simulink model "SF104A_MotCurrRegCfg"  (R2013b)
settings: Solver=FixedStepDiscrete  SolverMode=SingleTasking  StartTime=0.0  StopTime=1  FixedStep=0.002  RelTol=1e-3
values from neighbouring files (symbols this model uses):
  ARCHGLBPRM_2MILLISEC_SEC_F32 = DataDict.Constant    [SF104A_MotCurrRegCfg_DataDict.m]
  ARCHGLBPRM_2PI_ULS_F32 = DataDict.Constant    [SF104A_MotCurrRegCfg_DataDict.m]
  ARCHGLBPRM_HALFSQRT3_ULS_F32 = DataDict.Constant    [SF104A_MotCurrRegCfg_DataDict.m]
  MotCurrRegCfgCtrlrDynGainVehSpdCutOff = DataDict.Calibration    [SF104A_MotCurrRegCfg_DataDict.m]
  MotCurrRegCfgCurrLoopSecOrderTrfFctEna = DataDict.Calibration    [SF104A_MotCurrRegCfg_DataDict.m]
  MotCurrRegCfgIntglGainSampleTi = DataDict.Calibration    [SF104A_MotCurrRegCfg_DataDict.m]
  MotCurrRegCfgMotAgCompuDly = DataDict.Calibration    [SF104A_MotCurrRegCfg_DataDict.m]
  MotCurrRegCfgMotClsdLoopBwDaxY = DataDict.Calibration    [SF104A_MotCurrRegCfg_DataDict.m]
  MotCurrRegCfgMotClsdLoopBwQaxY = DataDict.Calibration    [SF104A_MotCurrRegCfg_DataDict.m]
  MotCurrRegCfgMotDampgRatDax = DataDict.Calibration    [SF104A_MotCurrRegCfg_DataDict.m]
  MotCurrRegCfgMotDampgRatQax = DataDict.Calibration    [SF104A_MotCurrRegCfg_DataDict.m]
  MotCurrRegCfgMotNatFrqDaxY = DataDict.Calibration    [SF104A_MotCurrRegCfg_DataDict.m]
  MotCurrRegCfgMotNatFrqQaxY = DataDict.Calibration    [SF104A_MotCurrRegCfg_DataDict.m]
  MotCurrRegCfgMotRVirtDax = DataDict.Calibration    [SF104A_MotCurrRegCfg_DataDict.m]
  MotCurrRegCfgMotRVirtQax = DataDict.Calibration    [SF104A_MotCurrRegCfg_DataDict.m]
  MOTDAMPGRATCON_ULS_F32 = DataDict.Constant    [SF104A_MotCurrRegCfg_DataDict.m]
  MotRefMdlFbCtrlDi = DataDict.ImprtdCal    [SF104A_MotCurrRegCfg_DataDict.m]
  POLETOPHA_ULS_F32 = DataDict.Constant    [SF104A_MotCurrRegCfg_DataDict.m]
  SysGlbPrmMotPoleCnt = DataDict.ImprtdCal    [SF104A_MotCurrRegCfg_DataDict.m]
  ZEROMOTCTRLGAIN_OHM_F32 = DataDict.Constant    [SF104A_MotCurrRegCfg_DataDict.m]
undefined symbols (not defined in the file or in its folder): MotCurrEolCalSt2
libraries: NxtrLim x11, FixdToFloat x4, LnrIntrpn x4, simulink x3, Fil x2, FloatToFixd x1
(part 2 of 3)

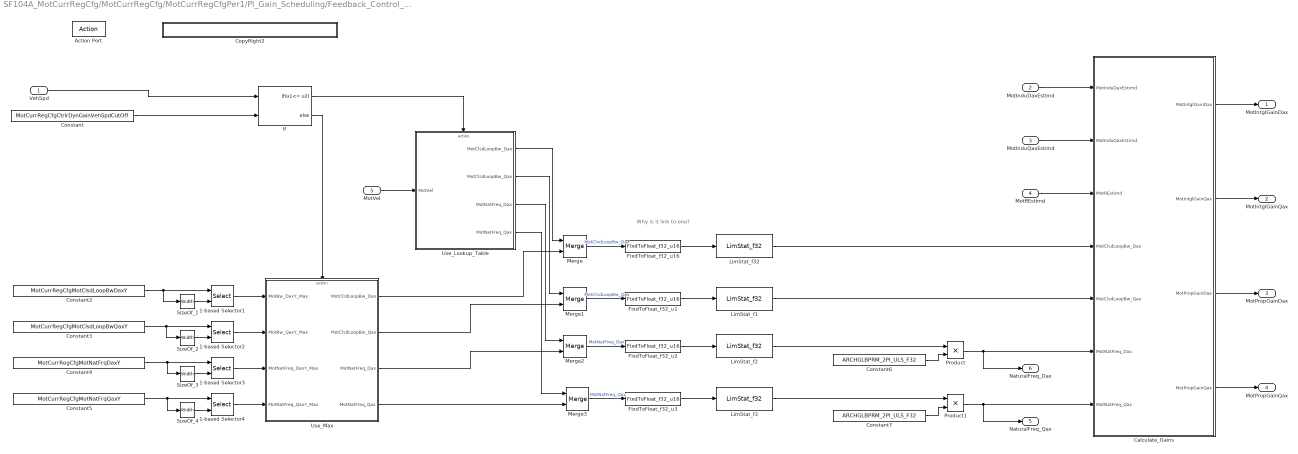
== system SF104A_MotCurrRegCfg/MotCurrRegCfg/MotCurrRegCfgPer1/PI_Gain_Scheduling/Feedback_Control_ Enabled ==
  note: Why is it link to one?
  VehSpd : Inport  RequirementInfo="{'linktype_rmi_doors' '0000bb43 (/E-STEER Core/SubSystem Specifications/Application Functions/SF99/SF104A Current Regulator Configuration)' '#SF104A_79' 'true' 'REQ:  SF104A_79' '' } %GIDa_d4012eee_a649_4ac2_87cc_e6d6b0b3897a"
  MotInduDaxEstimd : Inport  Port=2
  MotInduQaxEstimd : Inport  Port=3
  MotREstimd : Inport  Port=4
  MotVel : Inport  Port=5
  Action Port : ActionPort  ActionType=else
  1-based Selector1 : Selector  RequirementInfo="{'linktype_rmi_doors' '0000bb43 (/E-STEER Core/SubSystem Specifications/Application Functions/SF99/SF104A Current Regulator Configuration)' '#SF104A_79' 'true' 'REQ:  SF104A_79' '' } %GIDa_589180ec_3502_4fb0_bcbd_283ed4baffb4"  IndexOptions=Index vector (port)  Indices=[1 3]  OutputSizes=1
  1-based Selector2 : Selector  RequirementInfo="{'linktype_rmi_doors' '0000bb43 (/E-STEER Core/SubSystem Specifications/Application Functions/SF99/SF104A Current Regulator Configuration)' '#SF104A_79' 'true' 'REQ:  SF104A_79' '' } %GIDa_407a2e01_fdd5_4bd9_81d6_0d5cf37eba6c"  IndexOptions=Index vector (port)  Indices=[1 3]  OutputSizes=1
  1-based Selector3 : Selector  RequirementInfo="{'linktype_rmi_doors' '0000bb43 (/E-STEER Core/SubSystem Specifications/Application Functions/SF99/SF104A Current Regulator Configuration)' '#SF104A_79' 'true' 'REQ:  SF104A_79' '' } %GIDa_682592dd_431f_4320_acc1_e53b32b2246e"  IndexOptions=Index vector (port)  Indices=[1 3]  OutputSizes=1
  1-based Selector4 : Selector  RequirementInfo="{'linktype_rmi_doors' '0000bb43 (/E-STEER Core/SubSystem Specifications/Application Functions/SF99/SF104A Current Regulator Configuration)' '#SF104A_79' 'true' 'REQ:  SF104A_79' '' } %GIDa_f36723ae_5dbe_4097_8c41_5bcb9ed4023c"  IndexOptions=Index vector (port)  Indices=[1 3]  OutputSizes=1
  Calculate_Gains : Subsystem
  Constant : Constant  RequirementInfo="{'linktype_rmi_doors' '0000bb43 (/E-STEER Core/SubSystem Specifications/Application Functions/SF99/SF104A Current Regulator Configuration)' '#SF104A_78' 'true' 'REQ:  SF104A_78' '' ; 'linktype_rmi_doors' '0000bb43 (/E-STEER Core/SubSystem Specifications/Application Functions/SF99/SF104A Current Regulator Configuration)' '#SF104A_79' 'true' 'REQ:  SF104A_79' '' } %GIDa_958b7c24_09c8_4828_a866_90831bf7cec9"  Value=MotCurrRegCfgCtrlrDynGainVehSpdCutOff
  Constant2 : Constant  RequirementInfo="{'linktype_rmi_doors' '0000bb43 (/E-STEER Core/SubSystem Specifications/Application Functions/SF99/SF104A Current Regulator Configuration)' '#SF104A_79' 'true' 'REQ:  SF104A_79' '' } %GIDa_c6d19c06_a239_4f1d_9090_8e55eb46cc49"  Value=MotCurrRegCfgMotClsdLoopBwDaxY
  Constant3 : Constant  RequirementInfo="{'linktype_rmi_doors' '0000bb43 (/E-STEER Core/SubSystem Specifications/Application Functions/SF99/SF104A Current Regulator Configuration)' '#SF104A_79' 'true' 'REQ:  SF104A_79' '' } %GIDa_c8184e20_a470_41b5_9de4_df8206d45247"  Value=MotCurrRegCfgMotClsdLoopBwQaxY
  Constant4 : Constant  RequirementInfo="{'linktype_rmi_doors' '0000bb43 (/E-STEER Core/SubSystem Specifications/Application Functions/SF99/SF104A Current Regulator Configuration)' '#SF104A_79' 'true' 'REQ:  SF104A_79' '' } %GIDa_936bd16a_dd57_47b2_b427_064699f5e422"  Value=MotCurrRegCfgMotNatFrqDaxY
  Constant5 : Constant  RequirementInfo="{'linktype_rmi_doors' '0000bb43 (/E-STEER Core/SubSystem Specifications/Application Functions/SF99/SF104A Current Regulator Configuration)' '#SF104A_79' 'true' 'REQ:  SF104A_79' '' } %GIDa_74c709f6_b02e_4d6d_83a0_731230ecb531"  Value=MotCurrRegCfgMotNatFrqQaxY
  Constant6 : Constant  RequirementInfo="{'linktype_rmi_doors' '0000bb43 (/E-STEER Core/SubSystem Specifications/Application Functions/SF99/SF104A Current Regulator Configuration)' '#SF104A_102' 'true' 'REQ:  SF104A_102' '' } %GIDa_b282edf1_703a_4aa4_ac64_8ed08260268d"  Value=ARCHGLBPRM_2PI_ULS_F32
  Constant7 : Constant  RequirementInfo="{'linktype_rmi_doors' '0000bb43 (/E-STEER Core/SubSystem Specifications/Application Functions/SF99/SF104A Current Regulator Configuration)' '#SF104A_102' 'true' 'REQ:  SF104A_102' '' } %GIDa_4256d3f3_42bf_446c_99fe_c2102f71585c"  Value=ARCHGLBPRM_2PI_ULS_F32
  CopyRight2 : Subsystem  Description=|  mask(Copyright Information){none=on}
      | Copyright info block.                                               
      |                                                                     
      | Place copyright information at the top of every subsystem in design.
      mask prompts: none "No parameters"
      mask help: Place copyright information at the top of every subsystem in design.
      mask Display:
      | NxtrConf = 'Nexteer Confidential';
      | 
      | sys = bdroot; %handle for the current model ("system")
      | first = get_param(sys,'Created');
      | if(isempty(first))
      |     first = datestr(now,'yyyy');
      | else
      |     first = first(end-3:end);  %year is last four digits
      | end
      | 
      | last = get_param(sys,'LastModifiedDate');
      | if isempty(last)
      |     last = datestr(now,'yyyy');
      | else
      |     last = last(end-3:end);
      | end
      | 
      | if strcmp(first,last)
      |     fprintf('%s -- Copyright %s Nexteer',NxtrConf,first)
      | else
      |     fprintf('%s -- %s%s- %s Nexteer',NxtrConf,char(169),first,last)
      | end
  FixdToFloat_f32_u1 : FixdToFloat/FixdToFloat_f32_u16  RequirementInfo="{'linktype_rmi_doors' '0000bb43 (/E-STEER Core/SubSystem Specifications/Application Functions/SF99/SF104A Current Regulator Configuration)' '#SF104A_80' 'true' 'REQ:  SF104A_80' '' } %GIDa_cdd56955_31d2_4d8a_a8b5_3422d07a9cc3"  Param1=6
  FixdToFloat_f32_u16 : FixdToFloat/FixdToFloat_f32_u16  RequirementInfo="{'linktype_rmi_doors' '0000bb43 (/E-STEER Core/SubSystem Specifications/Application Functions/SF99/SF104A Current Regulator Configuration)' '#SF104A_80' 'true' 'REQ:  SF104A_80' '' } %GIDa_f1b66ba1_8dba_40d4_86dd_996fa52edd7e"  Param1=6
  FixdToFloat_f32_u2 : FixdToFloat/FixdToFloat_f32_u16  RequirementInfo="{'linktype_rmi_doors' '0000bb43 (/E-STEER Core/SubSystem Specifications/Application Functions/SF99/SF104A Current Regulator Configuration)' '#SF104A_80' 'true' 'REQ:  SF104A_80' '' } %GIDa_b2e93a0d_5c3b_4c50_809e_c273a336214e"  Param1=7
  FixdToFloat_f32_u3 : FixdToFloat/FixdToFloat_f32_u16  RequirementInfo="{'linktype_rmi_doors' '0000bb43 (/E-STEER Core/SubSystem Specifications/Application Functions/SF99/SF104A Current Regulator Configuration)' '#SF104A_80' 'true' 'REQ:  SF104A_80' '' } %GIDa_d0090763_1e7f_40a2_965a_24601edd0d3b"  Param1=7
  If : If  RequirementInfo="{'linktype_rmi_doors' '0000bb43 (/E-STEER Core/SubSystem Specifications/Application Functions/SF99/SF104A Current Regulator Configuration)' '#SF104A_79' 'true' 'REQ:  SF104A_79' '' } %GIDa_f82bf75b_6a97_4ea4_8f3d_8033f64935ce"  NumInputs=2  IfExpression=u1<= u2
  LimStat_f1 : NxtrLim/LimStat_f32  RequirementInfo="{'linktype_rmi_doors' '0000bb43 (/E-STEER Core/SubSystem Specifications/Application Functions/SF99/SF104A Current Regulator Configuration)' '#SF104A_80' 'true' 'REQ:  SF104A_80' '' } %GIDa_3cecd6ad_32cc_4b1f_aa10_fcdb0c715f80"  LoLim=CLSDLOOPBWLOLIM_HZ_F32  HiLim=CLSDLOOPBWHILIM_HZ_F32
      settings: AttributesFormatString=|
      | Low Limit: %<LoLim>
      | High Limit:%<HiLim>
  LimStat_f2 : NxtrLim/LimStat_f32  RequirementInfo="{'linktype_rmi_doors' '0000bb43 (/E-STEER Core/SubSystem Specifications/Application Functions/SF99/SF104A Current Regulator Configuration)' '#SF104A_81' 'true' 'REQ:  SF104A_81' '' } %GIDa_36a4b465_8351_4e04_b819_0dc46c43bdc9"  LoLim=MOTNATFREQLOLIM_HZ_F32  HiLim=MOTNATFREQHILIM_HZ_F32
      settings: AttributesFormatString=|
      | Low Limit: %<LoLim>
      | High Limit:%<HiLim>
  LimStat_f3 : NxtrLim/LimStat_f32  RequirementInfo="{'linktype_rmi_doors' '0000bb43 (/E-STEER Core/SubSystem Specifications/Application Functions/SF99/SF104A Current Regulator Configuration)' '#SF104A_81' 'true' 'REQ:  SF104A_81' '' } %GIDa_9ed236cb_3b1f_490e_9ae7_2fd3135aea91"  LoLim=MOTNATFREQLOLIM_HZ_F32  HiLim=MOTNATFREQHILIM_HZ_F32
      settings: AttributesFormatString=|
      | Low Limit: %<LoLim>
      | High Limit:%<HiLim>
  LimStat_f32 : NxtrLim/LimStat_f32  RequirementInfo="{'linktype_rmi_doors' '0000bb43 (/E-STEER Core/SubSystem Specifications/Application Functions/SF99/SF104A Current Regulator Configuration)' '#SF104A_80' 'true' 'REQ:  SF104A_80' '' } %GIDa_deaae8fa_c053_4079_930d_ea564ba246ac"  LoLim=CLSDLOOPBWLOLIM_HZ_F32  HiLim=CLSDLOOPBWHILIM_HZ_F32
      settings: AttributesFormatString=|
      | Low Limit: %<LoLim>
      | High Limit:%<HiLim>
  Merge{,1..3} (4 alike) : Merge
  Product : Product  RequirementInfo="{'linktype_rmi_doors' '0000bb43 (/E-STEER Core/SubSystem Specifications/Application Functions/SF99/SF104A Current Regulator Configuration)' '#SF104A_102' 'true' 'REQ:  SF104A_102' '' } %GIDa_3cd0d002_6bda_4754_8a91_ac567ffd6fcf"
  Product1 : Product  RequirementInfo="{'linktype_rmi_doors' '0000bb43 (/E-STEER Core/SubSystem Specifications/Application Functions/SF99/SF104A Current Regulator Configuration)' '#SF104A_102' 'true' 'REQ:  SF104A_102' '' } %GIDa_bc381f7c_753e_4b7a_a17b_9e8272c7f5b5"
  SizeOf_1 : Width  RequirementInfo="{'linktype_rmi_doors' '0000bb43 (/E-STEER Core/SubSystem Specifications/Application Functions/SF99/SF104A Current Regulator Configuration)' '#SF104A_79' 'true' 'REQ:  SF104A_79' '' } %GIDa_4fa22dab_14f6_4711_820b_245d3df30989"
  SizeOf_2 : Width  RequirementInfo="{'linktype_rmi_doors' '0000bb43 (/E-STEER Core/SubSystem Specifications/Application Functions/SF99/SF104A Current Regulator Configuration)' '#SF104A_79' 'true' 'REQ:  SF104A_79' '' } %GIDa_f85203f8_9228_43f4_adcd_ef2b2ee9324a"
  SizeOf_3 : Width  RequirementInfo="{'linktype_rmi_doors' '0000bb43 (/E-STEER Core/SubSystem Specifications/Application Functions/SF99/SF104A Current Regulator Configuration)' '#SF104A_79' 'true' 'REQ:  SF104A_79' '' } %GIDa_7aec3032_db38_4c0b_8b26_007f313a80fb"
  SizeOf_4 : Width  RequirementInfo="{'linktype_rmi_doors' '0000bb43 (/E-STEER Core/SubSystem Specifications/Application Functions/SF99/SF104A Current Regulator Configuration)' '#SF104A_79' 'true' 'REQ:  SF104A_79' '' } %GIDa_8d50dec5_beca_4d14_bba7_94989fd329f9"
  Use_Lookup_Table : Subsystem  RequirementInfo="{'linktype_rmi_doors' '0000bb43 (/E-STEER Core/SubSystem Specifications/Application Functions/SF99/SF104A Current Regulator Configuration)' '#SF104A_77' 'true' 'REQ:  SF104A_77' '' ; 'linktype_rmi_doors' '0000bb43 (/E-STEER Core/SubSystem Specifications/Application Functions/SF99/SF104A Current Regulator Configuration)' '#SF104A_78' 'true' 'REQ:  SF104A_78' '' } %GIDa_e9922d81_32a9_4035_8f98_a70368f4a8de"  TreatAsAtomicUnit=on
  Use_Max : Subsystem  RequirementInfo="{'linktype_rmi_doors' '0000bb43 (/E-STEER Core/SubSystem Specifications/Application Functions/SF99/SF104A Current Regulator Configuration)' '#SF104A_79' 'true' 'REQ:  SF104A_79' '' } %GIDa_22edcf58_3a45_4728_bcee_9fd3be778dd4"  TreatAsAtomicUnit=on
      settings: AttributesFormatString=pass_thru
  MotIntglGainDax : Outport
  MotIntglGainQax : Outport  Port=2
  MotPropGainDax : Outport  Port=3
  MotPropGainQax : Outport  Port=4
  NaturalFreq_Qax : Outport  Port=5
  NaturalFreq_Dax : Outport  Port=6
  wires:
  VehSpd/1 -> If/1
  Constant/1 -> If/2
  If/1 -> Use_Lookup_Table/Action
  If/2 -> Use_Max/Action
  MotVel/1 -> Use_Lookup_Table/1(MotVel)
  Use_Lookup_Table/1(MotClsdLoopBw_Dax) -> Merge/1
  Use_Lookup_Table/2(MotClsdLoopBw_Qax) -> Merge1/1
  Use_Lookup_Table/3(MotNatFreq_Dax) -> Merge2/1
  Use_Lookup_Table/4(MotNatFreq_Qax) -> Merge3/1
  Merge/1 -> FixdToFloat_f32_u16/1  "MotClsdLoopBw_Dax"
  Merge1/1 -> FixdToFloat_f32_u1/1  "MotClsdLoopBw_Qax"
  Merge2/1 -> FixdToFloat_f32_u2/1  "MotNatFreq_Dax"
  Merge3/1 -> FixdToFloat_f32_u3/1  "MotNatFreq_Qax"
  Constant6/1 -> Product/2
  Constant7/1 -> Product1/2
  Product/1 -> NaturalFreq_Dax/1, Calculate_Gains/6(MotNatFreq_Dax)
  Product1/1 -> NaturalFreq_Qax/1, Calculate_Gains/7(MotNatFreq_Qax)
  LimStat_f32/1 -> Calculate_Gains/4(MotClsdLoopBw_Dax)
  LimStat_f1/1 -> Calculate_Gains/5(MotClsdLoopBw_Qax)
  LimStat_f2/1 -> Product/1
  LimStat_f3/1 -> Product1/1
  Calculate_Gains/1(MotIntglGainDax) -> MotIntglGainDax/1
  Calculate_Gains/2(MotIntglGainQax) -> MotIntglGainQax/1
  Calculate_Gains/4(MotPropGainQax) -> MotPropGainQax/1
  Calculate_Gains/3(MotPropGainDax) -> MotPropGainDax/1
  MotREstimd/1 -> Calculate_Gains/3(MotREstimd)
  MotInduQaxEstimd/1 -> Calculate_Gains/2(MotInduQaxEstimd)
  MotInduDaxEstimd/1 -> Calculate_Gains/1(MotInduDaxEstimd)
  Use_Max/1(MotClsdLoopBw_Dax) -> Merge/2
  Use_Max/2(MotClsdLoopBw_Qax) -> Merge1/2
  Use_Max/3(MotNatFreq_Dax) -> Merge2/2
  Use_Max/4(MotNatFreq_Qax) -> Merge3/2
  Constant2/1 -> SizeOf_1/1, 1-based Selector1/1
  Constant3/1 -> SizeOf_2/1, 1-based Selector2/1
  Constant4/1 -> SizeOf_3/1, 1-based Selector3/1
  Constant5/1 -> SizeOf_4/1, 1-based Selector4/1
  1-based Selector1/1 -> Use_Max/1(MotBw_DaxY_Max)
  1-based Selector2/1 -> Use_Max/2(MotBw_QaxY_Max)
  1-based Selector3/1 -> Use_Max/3(MotNatFreq_DaxY_Max)
  1-based Selector4/1 -> Use_Max/4(MotNatFreq_QaxY_Max)
  FixdToFloat_f32_u16/1 -> LimStat_f32/1
  FixdToFloat_f32_u1/1 -> LimStat_f1/1
  FixdToFloat_f32_u2/1 -> LimStat_f2/1
  FixdToFloat_f32_u3/1 -> LimStat_f3/1
  SizeOf_1/1 -> 1-based Selector1/2
  SizeOf_2/1 -> 1-based Selector2/2
  SizeOf_3/1 -> 1-based Selector3/2
  SizeOf_4/1 -> 1-based Selector4/2

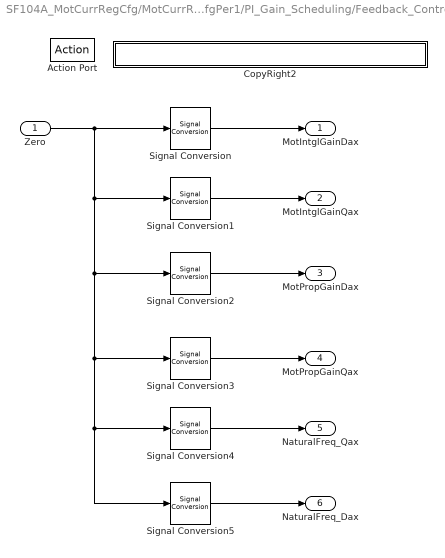
== system SF104A_MotCurrRegCfg/MotCurrRegCfg/MotCurrRegCfgPer1/PI_Gain_Scheduling/Feedback_Control_Disabled ==
  Zero : Inport  RequirementInfo="{'linktype_rmi_doors' '0000bb43 (/E-STEER Core/SubSystem Specifications/Application Functions/SF99/SF104A Current Regulator Configuration)' '#SF104A_85' 'true' 'REQ:  SF104A_85' '' } %GIDa_ac86b7b0_6f22_4db4_bc28_b14b0efc9a5a"
  Action Port : ActionPort  ActionType=then
  CopyRight2 : Subsystem  Description=|  mask(Copyright Information){none=on}
      | Copyright info block.                                               
      |                                                                     
      | Place copyright information at the top of every subsystem in design.
      mask prompts: none "No parameters"
      mask help: Place copyright information at the top of every subsystem in design.
      mask Display:
      | NxtrConf = 'Nexteer Confidential';
      | 
      | sys = bdroot; %handle for the current model ("system")
      | first = get_param(sys,'Created');
      | if(isempty(first))
      |     first = datestr(now,'yyyy');
      | else
      |     first = first(end-3:end);  %year is last four digits
      | end
      | 
      | last = get_param(sys,'LastModifiedDate');
      | if isempty(last)
      |     last = datestr(now,'yyyy');
      | else
      |     last = last(end-3:end);
      | end
      | 
      | if strcmp(first,last)
      |     fprintf('%s -- Copyright %s Nexteer',NxtrConf,first)
      | else
      |     fprintf('%s -- %s%s- %s Nexteer',NxtrConf,char(169),first,last)
      | end
  Signal Conversion : SignalConversion  RequirementInfo="{'linktype_rmi_doors' '0000bb43 (/E-STEER Core/SubSystem Specifications/Application Functions/SF99/SF104A Current Regulator Configuration)' '#SF104A_85' 'true' 'REQ:  SF104A_85' '' } %GIDa_3db586fd_44ec_407a_bf68_dc7beca2a271"
  Signal Conversion1 : SignalConversion  RequirementInfo="{'linktype_rmi_doors' '0000bb43 (/E-STEER Core/SubSystem Specifications/Application Functions/SF99/SF104A Current Regulator Configuration)' '#SF104A_85' 'true' 'REQ:  SF104A_85' '' } %GIDa_a8d76f7e_6ee4_43c8_b314_2be5e31a14f1"
  Signal Conversion2 : SignalConversion  RequirementInfo="{'linktype_rmi_doors' '0000bb43 (/E-STEER Core/SubSystem Specifications/Application Functions/SF99/SF104A Current Regulator Configuration)' '#SF104A_85' 'true' 'REQ:  SF104A_85' '' } %GIDa_09ae69bd_1d2f_4f7b_930a_4b035667f045"
  Signal Conversion3 : SignalConversion  RequirementInfo="{'linktype_rmi_doors' '0000bb43 (/E-STEER Core/SubSystem Specifications/Application Functions/SF99/SF104A Current Regulator Configuration)' '#SF104A_85' 'true' 'REQ:  SF104A_85' '' } %GIDa_ca777520_ed80_4f8d_b317_e0c5e258b136"
  Signal Conversion4 : SignalConversion  RequirementInfo="{'linktype_rmi_doors' '0000bb43 (/E-STEER Core/SubSystem Specifications/Application Functions/SF99/SF104A Current Regulator Configuration)' '#SF104A_85' 'true' 'REQ:  SF104A_85' '' } %GIDa_abd55f50_814d_4f33_95a4_f9dbf353d95e"
  Signal Conversion5 : SignalConversion  RequirementInfo="{'linktype_rmi_doors' '0000bb43 (/E-STEER Core/SubSystem Specifications/Application Functions/SF99/SF104A Current Regulator Configuration)' '#SF104A_85' 'true' 'REQ:  SF104A_85' '' } %GIDa_4a34024b_6912_4c83_9f6f_381b963a820d"
  MotIntglGainDax : Outport  RequirementInfo="{'linktype_rmi_doors' '0000bb43 (/E-STEER Core/SubSystem Specifications/Application Functions/SF99/SF104A Current Regulator Configuration)' '#SF104A_85' 'true' 'REQ:  SF104A_85' '' } %GIDa_1aaaa7a1_dc5e_4133_8033_4b32307ab873"
  MotIntglGainQax : Outport  RequirementInfo="{'linktype_rmi_doors' '0000bb43 (/E-STEER Core/SubSystem Specifications/Application Functions/SF99/SF104A Current Regulator Configuration)' '#SF104A_85' 'true' 'REQ:  SF104A_85' '' } %GIDa_ec0bc4d2_dc9c_44ff_971b_9e359e22d6d6"  Port=2
  MotPropGainDax : Outport  RequirementInfo="{'linktype_rmi_doors' '0000bb43 (/E-STEER Core/SubSystem Specifications/Application Functions/SF99/SF104A Current Regulator Configuration)' '#SF104A_85' 'true' 'REQ:  SF104A_85' '' } %GIDa_7463e1ab_8dee_4db6_97ae_176ec16a826a"  Port=3
  MotPropGainQax : Outport  RequirementInfo="{'linktype_rmi_doors' '0000bb43 (/E-STEER Core/SubSystem Specifications/Application Functions/SF99/SF104A Current Regulator Configuration)' '#SF104A_85' 'true' 'REQ:  SF104A_85' '' } %GIDa_b804823b_c4da_4f5f_a04e_3e5367f68e74"  Port=4
  NaturalFreq_Qax : Outport  Port=5
  NaturalFreq_Dax : Outport  Port=6
  wires:
  Zero/1 -> Signal Conversion2/1, Signal Conversion5/1, Signal Conversion4/1, Signal Conversion3/1, Signal Conversion1/1, Signal Conversion/1
  Signal Conversion/1 -> MotIntglGainDax/1
  Signal Conversion1/1 -> MotIntglGainQax/1
  Signal Conversion2/1 -> MotPropGainDax/1
  Signal Conversion3/1 -> MotPropGainQax/1
  Signal Conversion4/1 -> NaturalFreq_Qax/1
  Signal Conversion5/1 -> NaturalFreq_Dax/1

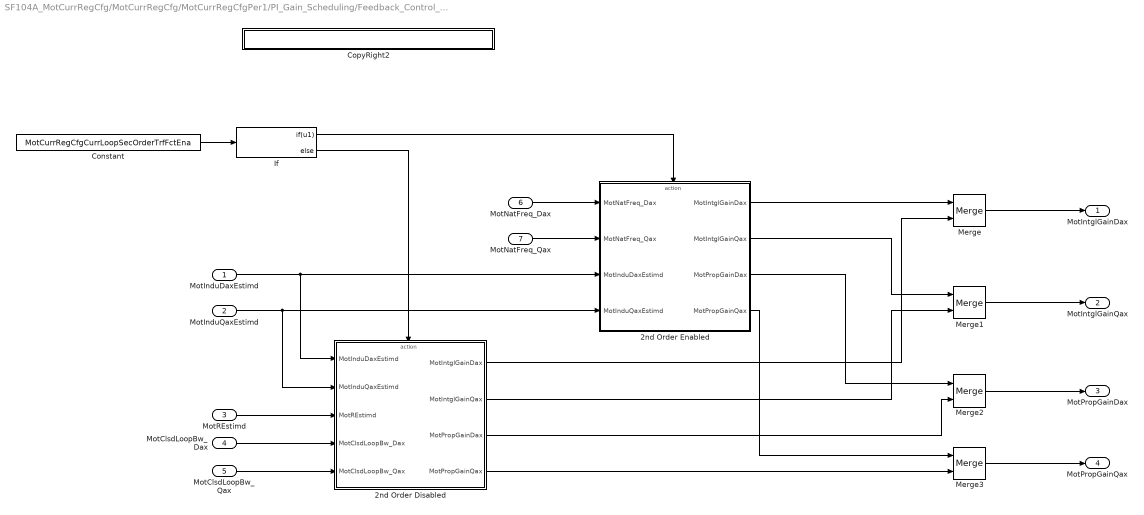
== system SF104A_MotCurrRegCfg/MotCurrRegCfg/MotCurrRegCfgPer1/PI_Gain_Scheduling/Feedback_Control_ Enabled/Calculate_Gains ==
  MotInduDaxEstimd : Inport
  MotInduQaxEstimd : Inport  Port=2
  MotREstimd : Inport  Port=3
  MotClsdLoopBw_Dax : Inport  Port=4
  MotClsdLoopBw_Qax : Inport  Port=5
  MotNatFreq_Dax : Inport  Port=6
  MotNatFreq_Qax : Inport  Port=7
  2nd Order Disabled : Subsystem  RequirementInfo="{'linktype_rmi_doors' '0000bb43 (/E-STEER Core/SubSystem Specifications/Application Functions/SF99/SF104A Current Regulator Configuration)' '#SF104A_88' 'true' 'REQ:  SF104A_88' '' } %GIDa_013f8656_5486_4d81_a93a_a7eac1d0f529"  TreatAsAtomicUnit=on
  2nd Order Enabled : Subsystem  RequirementInfo="{'linktype_rmi_doors' '0000bb43 (/E-STEER Core/SubSystem Specifications/Application Functions/SF99/SF104A Current Regulator Configuration)' '#SF104A_102' 'true' 'REQ:  SF104A_102' '' } %GIDa_23c422d9_6d41_4214_aeb0_c191b9bf3ca4"  TreatAsAtomicUnit=on
  Constant : Constant  RequirementInfo="{'linktype_rmi_doors' '0000bb43 (/E-STEER Core/SubSystem Specifications/Application Functions/SF99/SF104A Current Regulator Configuration)' '#SF104A_86' 'true' 'REQ:  SF104A_86' '' } %GIDa_e137901e_3c0a_47f7_9688_d8859e5a83bb"  Value=MotCurrRegCfgCurrLoopSecOrderTrfFctEna
  CopyRight2 : Subsystem  Description=|  mask(Copyright Information){none=on}
      | Copyright info block.                                               
      |                                                                     
      | Place copyright information at the top of every subsystem in design.
      mask prompts: none "No parameters"
      mask help: Place copyright information at the top of every subsystem in design.
      mask Display:
      | NxtrConf = 'Nexteer Confidential';
      | 
      | sys = bdroot; %handle for the current model ("system")
      | first = get_param(sys,'Created');
      | if(isempty(first))
      |     first = datestr(now,'yyyy');
      | else
      |     first = first(end-3:end);  %year is last four digits
      | end
      | 
      | last = get_param(sys,'LastModifiedDate');
      | if isempty(last)
      |     last = datestr(now,'yyyy');
      | else
      |     last = last(end-3:end);
      | end
      | 
      | if strcmp(first,last)
      |     fprintf('%s -- Copyright %s Nexteer',NxtrConf,first)
      | else
      |     fprintf('%s -- %s%s- %s Nexteer',NxtrConf,char(169),first,last)
      | end
  If : If  RequirementInfo="{'linktype_rmi_doors' '0000bb43 (/E-STEER Core/SubSystem Specifications/Application Functions/SF99/SF104A Current Regulator Configuration)' '#SF104A_102' 'true' 'REQ:  SF104A_102' '' ; 'linktype_rmi_doors' '0000bb43 (/E-STEER Core/SubSystem Specifications/Application Functions/SF99/SF104A Current Regulator Configuration)' '#SF104A_88' 'true' 'REQ:  SF104A_88' '' } %GIDa_b5fc30ee_ce16_4044_ada9_1cbb13591638"  IfExpression=u1
  Merge{,1..3} (4 alike) : Merge
  MotIntglGainDax : Outport
  MotIntglGainQax : Outport  Port=2
  MotPropGainDax : Outport  Port=3
  MotPropGainQax : Outport  Port=4
  wires:
  Constant/1 -> If/1
  If/2 -> 2nd Order Disabled/Action
  If/1 -> 2nd Order Enabled/Action
  MotClsdLoopBw_Qax/1 -> 2nd Order Disabled/5(MotClsdLoopBw_Qax)
  MotClsdLoopBw_Dax/1 -> 2nd Order Disabled/4(MotClsdLoopBw_Dax)
  MotInduQaxEstimd/1 -> 2nd Order Enabled/4(MotInduQaxEstimd), 2nd Order Disabled/2(MotInduQaxEstimd)
  MotREstimd/1 -> 2nd Order Disabled/3(MotREstimd)
  MotInduDaxEstimd/1 -> 2nd Order Enabled/3(MotInduDaxEstimd), 2nd Order Disabled/1(MotInduDaxEstimd)
  MotNatFreq_Dax/1 -> 2nd Order Enabled/1(MotNatFreq_Dax)
  MotNatFreq_Qax/1 -> 2nd Order Enabled/2(MotNatFreq_Qax)
  Merge/1 -> MotIntglGainDax/1
  Merge1/1 -> MotIntglGainQax/1
  Merge2/1 -> MotPropGainDax/1
  Merge3/1 -> MotPropGainQax/1
  2nd Order Enabled/1(MotIntglGainDax) -> Merge/1
  2nd Order Disabled/1(MotIntglGainDax) -> Merge/2
  2nd Order Enabled/2(MotIntglGainQax) -> Merge1/1
  2nd Order Disabled/2(MotIntglGainQax) -> Merge1/2
  2nd Order Enabled/3(MotPropGainDax) -> Merge2/1
  2nd Order Disabled/3(MotPropGainDax) -> Merge2/2
  2nd Order Enabled/4(MotPropGainQax) -> Merge3/1
  2nd Order Disabled/4(MotPropGainQax) -> Merge3/2

== system SF104A_MotCurrRegCfg/MotCurrRegCfg/MotCurrRegCfgPer1/PI_Gain_Scheduling/Feedback_Control_ Enabled/CopyRight2 ==

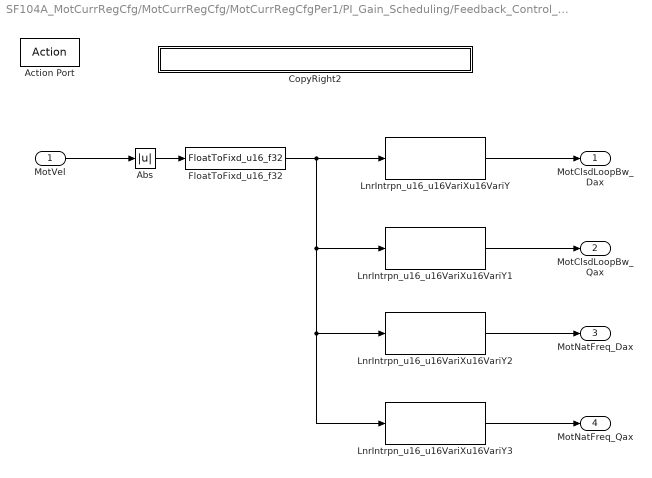
== system SF104A_MotCurrRegCfg/MotCurrRegCfg/MotCurrRegCfgPer1/PI_Gain_Scheduling/Feedback_Control_ Enabled/Use_Lookup_Table ==
  MotVel : Inport  RequirementInfo="{'linktype_rmi_doors' '0000bb43 (/E-STEER Core/SubSystem Specifications/Application Functions/SF99/SF104A Current Regulator Configuration)' '#SF104A_76' 'true' 'REQ:  SF104A_76' '' ; 'linktype_rmi_doors' '0000bb43 (/E-STEER Core/SubSystem Specifications/Application Functions/SF99/SF104A Current Regulator Configuration)' '#SF104A_77' 'true' 'REQ:  SF104A_77' '' } %GIDa_ed976189_f55e_4a06_b7f6_ea121c20981a"
  Action Port : ActionPort  ActionType=then
  Abs : Abs  RequirementInfo="{'linktype_rmi_doors' '0000bb43 (/E-STEER Core/SubSystem Specifications/Application Functions/SF99/SF104A Current Regulator Configuration)' '#SF104A_76' 'true' 'REQ:  SF104A_76' '' } %GIDa_b9887098_5366_4f75_9d5b_f45e8325f200"
  CopyRight2 : Subsystem  Description=|  mask(Copyright Information){none=on}
      | Copyright info block.                                               
      |                                                                     
      | Place copyright information at the top of every subsystem in design.
      mask prompts: none "No parameters"
      mask help: Place copyright information at the top of every subsystem in design.
      mask Display:
      | NxtrConf = 'Nexteer Confidential';
      | 
      | sys = bdroot; %handle for the current model ("system")
      | first = get_param(sys,'Created');
      | if(isempty(first))
      |     first = datestr(now,'yyyy');
      | else
      |     first = first(end-3:end);  %year is last four digits
      | end
      | 
      | last = get_param(sys,'LastModifiedDate');
      | if isempty(last)
      |     last = datestr(now,'yyyy');
      | else
      |     last = last(end-3:end);
      | end
      | 
      | if strcmp(first,last)
      |     fprintf('%s -- Copyright %s Nexteer',NxtrConf,first)
      | else
      |     fprintf('%s -- %s%s- %s Nexteer',NxtrConf,char(169),first,last)
      | end
  FloatToFixd_u16_f32 : FloatToFixd/FloatToFixd_u16_f32  RequirementInfo="{'linktype_rmi_doors' '0000bb43 (/E-STEER Core/SubSystem Specifications/Application Functions/SF99/SF104A Current Regulator Configuration)' '#SF104A_76' 'true' 'REQ:  SF104A_76' '' } %GIDa_16084c7b_ab98_4db5_b1e7_8fa9575a8448"  Param1=5
  LnrIntrpn_u16_u16VariXu16VariY : LnrIntrpn/LnrIntrpn_u16_u16VariXu16VariY  RequirementInfo="{'linktype_rmi_doors' '0000bb43 (/E-STEER Core/SubSystem Specifications/Application Functions/SF99/SF104A Current Regulator Configuration)' '#SF104A_76' 'true' 'REQ:  SF104A_76' '' } %GIDa_616b0792_308c_4259_827b_b463a69d75c5"  XTbl=MotCurrRegCfgMotCtrlPrmSelnX  YTbl=MotCurrRegCfgMotClsdLoopBwDaxY
      settings: AttributesFormatString=Lnr ( u16VariX , u16VariY )
  LnrIntrpn_u16_u16VariXu16VariY1 : LnrIntrpn/LnrIntrpn_u16_u16VariXu16VariY  RequirementInfo="{'linktype_rmi_doors' '0000bb43 (/E-STEER Core/SubSystem Specifications/Application Functions/SF99/SF104A Current Regulator Configuration)' '#SF104A_76' 'true' 'REQ:  SF104A_76' '' } %GIDa_3ac12756_c50f_40e0_ad71_8a239043b205"  XTbl=MotCurrRegCfgMotCtrlPrmSelnX  YTbl=MotCurrRegCfgMotClsdLoopBwQaxY
      settings: AttributesFormatString=Lnr ( u16VariX , u16VariY )
  LnrIntrpn_u16_u16VariXu16VariY2 : LnrIntrpn/LnrIntrpn_u16_u16VariXu16VariY  RequirementInfo="{'linktype_rmi_doors' '0000bb43 (/E-STEER Core/SubSystem Specifications/Application Functions/SF99/SF104A Current Regulator Configuration)' '#SF104A_77' 'true' 'REQ:  SF104A_77' '' } %GIDa_4422ee51_6f48_459f_976a_0b86c3ed4c22"  XTbl=MotCurrRegCfgMotCtrlPrmSelnX  YTbl=MotCurrRegCfgMotNatFrqDaxY
      settings: AttributesFormatString=Lnr ( u16VariX , u16VariY )
  LnrIntrpn_u16_u16VariXu16VariY3 : LnrIntrpn/LnrIntrpn_u16_u16VariXu16VariY  RequirementInfo="{'linktype_rmi_doors' '0000bb43 (/E-STEER Core/SubSystem Specifications/Application Functions/SF99/SF104A Current Regulator Configuration)' '#SF104A_77' 'true' 'REQ:  SF104A_77' '' } %GIDa_426c7479_e669_4515_bcad_b7626b0e0fb9"  XTbl=MotCurrRegCfgMotCtrlPrmSelnX  YTbl=MotCurrRegCfgMotNatFrqQaxY
      settings: AttributesFormatString=Lnr ( u16VariX , u16VariY )
  MotClsdLoopBw_Dax : Outport  RequirementInfo="{'linktype_rmi_doors' '0000bb43 (/E-STEER Core/SubSystem Specifications/Application Functions/SF99/SF104A Current Regulator Configuration)' '#SF104A_76' 'true' 'REQ:  SF104A_76' '' } %GIDa_cd97627e_bb1a_4496_a663_03b1d08b4a46"
  MotClsdLoopBw_Qax : Outport  RequirementInfo="{'linktype_rmi_doors' '0000bb43 (/E-STEER Core/SubSystem Specifications/Application Functions/SF99/SF104A Current Regulator Configuration)' '#SF104A_76' 'true' 'REQ:  SF104A_76' '' } %GIDa_5f5d3292_e4b0_4f00_ad72_6592f02510f7"  Port=2
  MotNatFreq_Dax : Outport  RequirementInfo="{'linktype_rmi_doors' '0000bb43 (/E-STEER Core/SubSystem Specifications/Application Functions/SF99/SF104A Current Regulator Configuration)' '#SF104A_77' 'true' 'REQ:  SF104A_77' '' } %GIDa_c0d855af_629c_4e42_ba67_5dc89bc24185"  Port=3
  MotNatFreq_Qax : Outport  RequirementInfo="{'linktype_rmi_doors' '0000bb43 (/E-STEER Core/SubSystem Specifications/Application Functions/SF99/SF104A Current Regulator Configuration)' '#SF104A_77' 'true' 'REQ:  SF104A_77' '' } %GIDa_8cd2fd4f_d3aa_4ad6_9dcb_c474b6f6311f"  Port=4
  wires:
  MotVel/1 -> Abs/1
  Abs/1 -> FloatToFixd_u16_f32/1
  FloatToFixd_u16_f32/1 -> LnrIntrpn_u16_u16VariXu16VariY1/1, LnrIntrpn_u16_u16VariXu16VariY2/1, LnrIntrpn_u16_u16VariXu16VariY3/1, LnrIntrpn_u16_u16VariXu16VariY/1
  LnrIntrpn_u16_u16VariXu16VariY/1 -> MotClsdLoopBw_Dax/1
  LnrIntrpn_u16_u16VariXu16VariY1/1 -> MotClsdLoopBw_Qax/1
  LnrIntrpn_u16_u16VariXu16VariY2/1 -> MotNatFreq_Dax/1
  LnrIntrpn_u16_u16VariXu16VariY3/1 -> MotNatFreq_Qax/1

== system SF104A_MotCurrRegCfg/MotCurrRegCfg/MotCurrRegCfgPer1/PI_Gain_Scheduling/Feedback_Control_ Enabled/Use_Max ==
  MotBw_DaxY_Max : Inport
  MotBw_QaxY_Max : Inport  Port=2
  MotNatFreq_DaxY_Max : Inport  Port=3
  MotNatFreq_QaxY_Max : Inport  Port=4
  Action Port : ActionPort  ActionType=else
  CopyRight2 : Subsystem  Description=|  mask(Copyright Information){none=on}
      | Copyright info block.                                               
      |                                                                     
      | Place copyright information at the top of every subsystem in design.
      mask prompts: none "No parameters"
      mask help: Place copyright information at the top of every subsystem in design.
      mask Display:
      | NxtrConf = 'Nexteer Confidential';
      | 
      | sys = bdroot; %handle for the current model ("system")
      | first = get_param(sys,'Created');
      | if(isempty(first))
      |     first = datestr(now,'yyyy');
      | else
      |     first = first(end-3:end);  %year is last four digits
      | end
      | 
      | last = get_param(sys,'LastModifiedDate');
      | if isempty(last)
      |     last = datestr(now,'yyyy');
      | else
      |     last = last(end-3:end);
      | end
      | 
      | if strcmp(first,last)
      |     fprintf('%s -- Copyright %s Nexteer',NxtrConf,first)
      | else
      |     fprintf('%s -- %s%s- %s Nexteer',NxtrConf,char(169),first,last)
      | end
  MotClsdLoopBw_Dax : Outport
  MotClsdLoopBw_Qax : Outport  Port=2
  MotNatFreq_Dax : Outport  Port=3
  MotNatFreq_Qax : Outport  Port=4
  wires:
  MotBw_DaxY_Max/1 -> MotClsdLoopBw_Dax/1
  MotBw_QaxY_Max/1 -> MotClsdLoopBw_Qax/1
  MotNatFreq_DaxY_Max/1 -> MotNatFreq_Dax/1
  MotNatFreq_QaxY_Max/1 -> MotNatFreq_Qax/1

== system SF104A_MotCurrRegCfg/MotCurrRegCfg/MotCurrRegCfgPer1/PI_Gain_Scheduling/Feedback_Control_Disabled/CopyRight2 ==

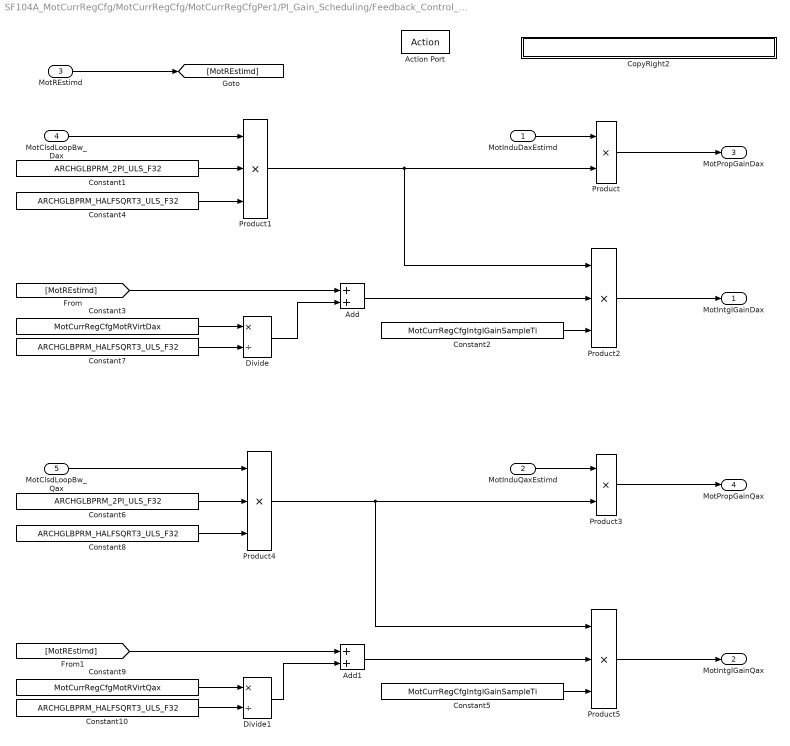
== system SF104A_MotCurrRegCfg/MotCurrRegCfg/MotCurrRegCfgPer1/PI_Gain_Scheduling/Feedback_Control_ Enabled/Calculate_Gains/2nd Order Disabled ==
  MotInduDaxEstimd : Inport  RequirementInfo="{'linktype_rmi_doors' '0000bb43 (/E-STEER Core/SubSystem Specifications/Application Functions/SF99/SF104A Current Regulator Configuration)' '#SF104A_88' 'true' 'REQ:  SF104A_88' '' } %GIDa_a0380e4d_6514_4d6c_b5c9_33cd68359e79"
  MotInduQaxEstimd : Inport  RequirementInfo="{'linktype_rmi_doors' '0000bb43 (/E-STEER Core/SubSystem Specifications/Application Functions/SF99/SF104A Current Regulator Configuration)' '#SF104A_88' 'true' 'REQ:  SF104A_88' '' } %GIDa_fa138374_a89e_4262_b9a2_5d706d1252b4"  Port=2
  MotREstimd : Inport  RequirementInfo="{'linktype_rmi_doors' '0000bb43 (/E-STEER Core/SubSystem Specifications/Application Functions/SF99/SF104A Current Regulator Configuration)' '#SF104A_88' 'true' 'REQ:  SF104A_88' '' } %GIDa_9f5f8e92_4fc0_4f81_9f90_7bb9bcd1a0cd"  Port=3
  MotClsdLoopBw_Dax : Inport  RequirementInfo="{'linktype_rmi_doors' '0000bb43 (/E-STEER Core/SubSystem Specifications/Application Functions/SF99/SF104A Current Regulator Configuration)' '#SF104A_88' 'true' 'REQ:  SF104A_88' '' } %GIDa_77129b9f_a7d6_42bf_9dfd_e8dc917c3c7a"  Port=4
  MotClsdLoopBw_Qax : Inport  RequirementInfo="{'linktype_rmi_doors' '0000bb43 (/E-STEER Core/SubSystem Specifications/Application Functions/SF99/SF104A Current Regulator Configuration)' '#SF104A_88' 'true' 'REQ:  SF104A_88' '' } %GIDa_0a04cf5f_bec3_44f2_90e8_108766046736"  Port=5
  Action Port : ActionPort  RequirementInfo={} %GIDa_f52aa930_ba25_449b_be45_377c57e7b084  ActionType=else
  Add : Sum  RequirementInfo="{'linktype_rmi_doors' '0000bb43 (/E-STEER Core/SubSystem Specifications/Application Functions/SF99/SF104A Current Regulator Configuration)' '#SF104A_88' 'true' 'REQ:  SF104A_88' '' } %GIDa_133e2e09_cf76_4bb4_91d6_bac496a66ea7"
  Add1 : Sum  RequirementInfo="{'linktype_rmi_doors' '0000bb43 (/E-STEER Core/SubSystem Specifications/Application Functions/SF99/SF104A Current Regulator Configuration)' '#SF104A_88' 'true' 'REQ:  SF104A_88' '' } %GIDa_1060c71f_d494_49ca_ab89_d92977cc6f00"
  Constant1 : Constant  RequirementInfo="{'linktype_rmi_doors' '0000bb43 (/E-STEER Core/SubSystem Specifications/Application Functions/SF99/SF104A Current Regulator Configuration)' '#SF104A_88' 'true' 'REQ:  SF104A_88' '' } %GIDa_8ab13d07_a842_4f2e_81b5_6b59de990e2a"  Value=ARCHGLBPRM_2PI_ULS_F32
  Constant10 : Constant  RequirementInfo="{'linktype_rmi_doors' '0000bb43 (/E-STEER Core/SubSystem Specifications/Application Functions/SF99/SF104A Current Regulator Configuration)' '#SF104A_88' 'true' 'REQ:  SF104A_88' '' } %GIDa_b61e4ccc_4bd4_4125_bd81_b940749f6018"  Value=ARCHGLBPRM_HALFSQRT3_ULS_F32
  Constant2 : Constant  RequirementInfo="{'linktype_rmi_doors' '0000bb43 (/E-STEER Core/SubSystem Specifications/Application Functions/SF99/SF104A Current Regulator Configuration)' '#SF104A_118' 'true' 'REQ:  SF104A_118' '' ; 'linktype_rmi_doors' '0000bb43 (/E-STEER Core/SubSystem Specifications/Application Functions/SF99/SF104A Current Regulator Configuration)' '#SF104A_102' 'true' 'REQ:  SF104A_102' '' } %GIDa_0372788a_13f9_4130_903e_6ee9f6e11ec2"  Value=MotCurrRegCfgIntglGainSampleTi
  Constant3 : Constant  RequirementInfo="{'linktype_rmi_doors' '0000bb43 (/E-STEER Core/SubSystem Specifications/Application Functions/SF99/SF104A Current Regulator Configuration)' '#SF104A_88' 'true' 'REQ:  SF104A_88' '' } %GIDa_445080f2_864b_4824_97ff_e7ba78646746"  Value=MotCurrRegCfgMotRVirtDax
  Constant4 : Constant  RequirementInfo="{'linktype_rmi_doors' '0000bb43 (/E-STEER Core/SubSystem Specifications/Application Functions/SF99/SF104A Current Regulator Configuration)' '#SF104A_88' 'true' 'REQ:  SF104A_88' '' } %GIDa_b0498fab_e0d7_4ad2_be9b_851d6e4abc37"  Value=ARCHGLBPRM_HALFSQRT3_ULS_F32
  Constant5 : Constant  RequirementInfo="{'linktype_rmi_doors' '0000bb43 (/E-STEER Core/SubSystem Specifications/Application Functions/SF99/SF104A Current Regulator Configuration)' '#SF104A_118' 'true' 'REQ:  SF104A_118' '' ; 'linktype_rmi_doors' '0000bb43 (/E-STEER Core/SubSystem Specifications/Application Functions/SF99/SF104A Current Regulator Configuration)' '#SF104A_102' 'true' 'REQ:  SF104A_102' '' } %GIDa_3bde522d_905e_4200_be3c_ef0a6f99362a"  Value=MotCurrRegCfgIntglGainSampleTi
  Constant6 : Constant  RequirementInfo="{'linktype_rmi_doors' '0000bb43 (/E-STEER Core/SubSystem Specifications/Application Functions/SF99/SF104A Current Regulator Configuration)' '#SF104A_88' 'true' 'REQ:  SF104A_88' '' } %GIDa_3876953e_8477_47fb_85db_9a39933b869e"  Value=ARCHGLBPRM_2PI_ULS_F32
  Constant7 : Constant  RequirementInfo="{'linktype_rmi_doors' '0000bb43 (/E-STEER Core/SubSystem Specifications/Application Functions/SF99/SF104A Current Regulator Configuration)' '#SF104A_88' 'true' 'REQ:  SF104A_88' '' } %GIDa_c237cb3e_bdf3_45d6_888e_840652958acf"  Value=ARCHGLBPRM_HALFSQRT3_ULS_F32
  Constant8 : Constant  RequirementInfo="{'linktype_rmi_doors' '0000bb43 (/E-STEER Core/SubSystem Specifications/Application Functions/SF99/SF104A Current Regulator Configuration)' '#SF104A_88' 'true' 'REQ:  SF104A_88' '' } %GIDa_c5331148_d4fd_4a25_b374_37dc68ddf89f"  Value=ARCHGLBPRM_HALFSQRT3_ULS_F32
  Constant9 : Constant  RequirementInfo="{'linktype_rmi_doors' '0000bb43 (/E-STEER Core/SubSystem Specifications/Application Functions/SF99/SF104A Current Regulator Configuration)' '#SF104A_88' 'true' 'REQ:  SF104A_88' '' } %GIDa_11c43035_c400_4c6f_a853_09fd1b99e0d1"  Value=MotCurrRegCfgMotRVirtQax
  CopyRight2 : Subsystem  Description=|  mask(Copyright Information){none=on}
      | Copyright info block.                                               
      |                                                                     
      | Place copyright information at the top of every subsystem in design.
      mask prompts: none "No parameters"
      mask help: Place copyright information at the top of every subsystem in design.
      mask Display:
      | NxtrConf = 'Nexteer Confidential';
      | 
      | sys = bdroot; %handle for the current model ("system")
      | first = get_param(sys,'Created');
      | if(isempty(first))
      |     first = datestr(now,'yyyy');
      | else
      |     first = first(end-3:end);  %year is last four digits
      | end
      | 
      | last = get_param(sys,'LastModifiedDate');
      | if isempty(last)
      |     last = datestr(now,'yyyy');
      | else
      |     last = last(end-3:end);
      | end
      | 
      | if strcmp(first,last)
      |     fprintf('%s -- Copyright %s Nexteer',NxtrConf,first)
      | else
      |     fprintf('%s -- %s%s- %s Nexteer',NxtrConf,char(169),first,last)
      | end
  Divide : Product  RequirementInfo="{'linktype_rmi_doors' '0000bb43 (/E-STEER Core/SubSystem Specifications/Application Functions/SF99/SF104A Current Regulator Configuration)' '#SF104A_88' 'true' 'REQ:  SF104A_88' '' } %GIDa_9543fc79_7cda_452b_970a_6569b528171b"  Inputs=*/
  Divide1 : Product  RequirementInfo="{'linktype_rmi_doors' '0000bb43 (/E-STEER Core/SubSystem Specifications/Application Functions/SF99/SF104A Current Regulator Configuration)' '#SF104A_88' 'true' 'REQ:  SF104A_88' '' } %GIDa_2f1ae7e0_9ce5_4d15_bb64_8d033b6a28a9"  Inputs=*/
  Product : Product  RequirementInfo="{'linktype_rmi_doors' '0000bb43 (/E-STEER Core/SubSystem Specifications/Application Functions/SF99/SF104A Current Regulator Configuration)' '#SF104A_88' 'true' 'REQ:  SF104A_88' '' } %GIDa_eef734f3_cd83_43ad_b75c_ceaed2cd9840"
  Product1 : Product  RequirementInfo="{'linktype_rmi_doors' '0000bb43 (/E-STEER Core/SubSystem Specifications/Application Functions/SF99/SF104A Current Regulator Configuration)' '#SF104A_88' 'true' 'REQ:  SF104A_88' '' } %GIDa_6039b0ee_8124_4565_868f_1754597c193d"  Inputs=3
  Product2 : Product  RequirementInfo="{'linktype_rmi_doors' '0000bb43 (/E-STEER Core/SubSystem Specifications/Application Functions/SF99/SF104A Current Regulator Configuration)' '#SF104A_118' 'true' 'REQ:  SF104A_118' '' ; 'linktype_rmi_doors' '0000bb43 (/E-STEER Core/SubSystem Specifications/Application Functions/SF99/SF104A Current Regulator Configuration)' '#SF104A_88' 'true' 'REQ:  SF104A_88' '' } %GIDa_82bb1531_e69c_43af_97e5_c626828bd751"  Inputs=3
  Product3 : Product  RequirementInfo="{'linktype_rmi_doors' '0000bb43 (/E-STEER Core/SubSystem Specifications/Application Functions/SF99/SF104A Current Regulator Configuration)' '#SF104A_88' 'true' 'REQ:  SF104A_88' '' } %GIDa_fa59358f_fe98_49b2_8812_a4bddd19c5d0"
  Product4 : Product  RequirementInfo="{'linktype_rmi_doors' '0000bb43 (/E-STEER Core/SubSystem Specifications/Application Functions/SF99/SF104A Current Regulator Configuration)' '#SF104A_88' 'true' 'REQ:  SF104A_88' '' } %GIDa_6acbc4d8_ff91_499d_a642_12495ad7aa5d"  Inputs=3
  Product5 : Product  RequirementInfo="{'linktype_rmi_doors' '0000bb43 (/E-STEER Core/SubSystem Specifications/Application Functions/SF99/SF104A Current Regulator Configuration)' '#SF104A_118' 'true' 'REQ:  SF104A_118' '' ; 'linktype_rmi_doors' '0000bb43 (/E-STEER Core/SubSystem Specifications/Application Functions/SF99/SF104A Current Regulator Configuration)' '#SF104A_88' 'true' 'REQ:  SF104A_88' '' } %GIDa_5808314d_73d3_4c41_ab14_c5bcd8407028"  Inputs=3
  MotIntglGainDax : Outport  RequirementInfo="{'linktype_rmi_doors' '0000bb43 (/E-STEER Core/SubSystem Specifications/Application Functions/SF99/SF104A Current Regulator Configuration)' '#SF104A_88' 'true' 'REQ:  SF104A_88' '' } %GIDa_5f4de269_8539_4d8f_822d_08871132d2d9"
  MotIntglGainQax : Outport  RequirementInfo="{'linktype_rmi_doors' '0000bb43 (/E-STEER Core/SubSystem Specifications/Application Functions/SF99/SF104A Current Regulator Configuration)' '#SF104A_88' 'true' 'REQ:  SF104A_88' '' } %GIDa_b7e3d09e_e4fa_4df2_90c7_f9dd7eb8e627"  Port=2
  MotPropGainDax : Outport  RequirementInfo="{'linktype_rmi_doors' '0000bb43 (/E-STEER Core/SubSystem Specifications/Application Functions/SF99/SF104A Current Regulator Configuration)' '#SF104A_88' 'true' 'REQ:  SF104A_88' '' } %GIDa_010db993_f3f2_4aca_b1c6_ece0db8b5f5d"  Port=3
  MotPropGainQax : Outport  RequirementInfo="{'linktype_rmi_doors' '0000bb43 (/E-STEER Core/SubSystem Specifications/Application Functions/SF99/SF104A Current Regulator Configuration)' '#SF104A_88' 'true' 'REQ:  SF104A_88' '' } %GIDa_998fb431_b393_4207_a158_d415ea3c2a59"  Port=4
  wires:
  Constant1/1 -> Product1/2
  MotClsdLoopBw_Dax/1 -> Product1/1
  Product1/1 -> Product/2, Product2/1
  Constant3/1 -> Divide/1
  Constant7/1 -> Divide/2
  Divide/1 -> Add/2
  Add/1 -> Product2/2
  Constant2/1 -> Product2/3
  Constant4/1 -> Product1/3
  Product/1 -> MotPropGainDax/1
  Product2/1 -> MotIntglGainDax/1
  MotREstimd/1 -> [MotREstimd]
  [MotREstimd] -> Add/1
  MotInduDaxEstimd/1 -> Product/1
  MotInduQaxEstimd/1 -> Product3/1
  MotClsdLoopBw_Qax/1 -> Product4/1
  Constant6/1 -> Product4/2
  Constant8/1 -> Product4/3
  Product4/1 -> Product5/1, Product3/2
  Constant5/1 -> Product5/3
  Constant9/1 -> Divide1/1
  Constant10/1 -> Divide1/2
  Divide1/1 -> Add1/2
  [MotREstimd] -> Add1/1
  Add1/1 -> Product5/2
  Product3/1 -> MotPropGainQax/1
  Product5/1 -> MotIntglGainQax/1
